simulink model "Demo2_1"  (R2016a)
settings: Solver=ode45  StartTime=0.0  StopTime=10  MaxStep=0.1  RelTol=1e-3
settings Model: Creator=peter  LastModifiedBy=peter
settings GRTTargetCC: GeneratePreprocessorConditionals=Use local settings

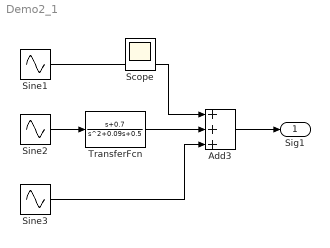
== system Demo2_1 ==
  Add3 : Sum  Inputs=+++
  Sine1 : Sin  Amplitude=0.1  Frequency=1.0472
  Sine2 : Sin  Amplitude=2
  Sine3 : Sin  Amplitude=0.3  Frequency=0.5236
  TransferFcn : TransferFcn  Numerator=[1, 0.7]  Denominator=[1, 0.09, 0.5]
  Sig1 : Outport
  Scope : Scope
  wires:
  Sine1/1 -> Add3/1
  Sine2/1 -> TransferFcn/1
  Sine3/1 -> Add3/3
  Add3/1 -> Sig1/1
  TransferFcn/1 -> Add3/2
